simulink model "Pendule_TrueTime_SA"  (R2020a)
settings: Solver=ode45  StartTime=0.0  StopTime=30  RelTol=1e-3  EnableMultiTasking=on
libraries: truetime x3
settings Model: ExtModeAutoUpdateStatusClock=off  Creator=anton  LastModifiedBy=Pierre
settings DataIOCC: LimitDataPoints=on  SaveFormat=Array  SignalLoggingSaveFormat=ModelDataLogs  ReturnWorkspaceOutputs=off
settings OptimizationCC: BooleanDataType=off  LifeSpan=inf
settings DebuggingCC: SaveWithParameterizedLinksMsg=none  UnderspecifiedInitializationDetection=Classic  MergeDetectMultiDrivingBlocksExec=none  SignalResolutionControl=TryResolveAllWithWarning  MultiTaskDSMMsg=warning  MultiTaskCondExecSysMsg=none  FcnCallInpInsideContextMsg=warning  SFUnexpectedBacktrackingDiag=warning  SFNoUnconditionalDefaultTransitionDiag=warning  SFExecutionAtInitializationDiag=none  ArithmeticOperatorsInVariantConditions=warning
settings HardwareCC: ProdBitPerPointer=32  ProdBitPerSizeT=32  ProdBitPerPtrDiffT=32  ProdLargestAtomicFloat=None  ProdIntDivRoundTo=Undefined  ProdEndianess=Unspecified  ProdWordSize=32  ProdHWDeviceType=32-bit Generic  TargetUnknown=on
settings ModelReferenceCC: PropagateSignalLabelsOutOfModel=off
settings SFSimCC: SimUseLocalCustomCode=off  CustomCodeUndefinedFunction=UseInterfaceOnly
settings RTWCC: RTWUseLocalCustomCode=off
settings CodeAppCC: StateflowObjectComments=on
settings GRTTargetCC: TargetLangStandard=C89/C90 (ANSI)  CombineOutputUpdateFcns=off  GRTInterface=on
settings ConfigComp: CovMetricSettings=dw  CovHtmlReporting=on  CovSaveCumulativeToWorkspaceVar=on  CovSaveSingleToWorkspaceVar=on  CovExternalEMLEnable=off

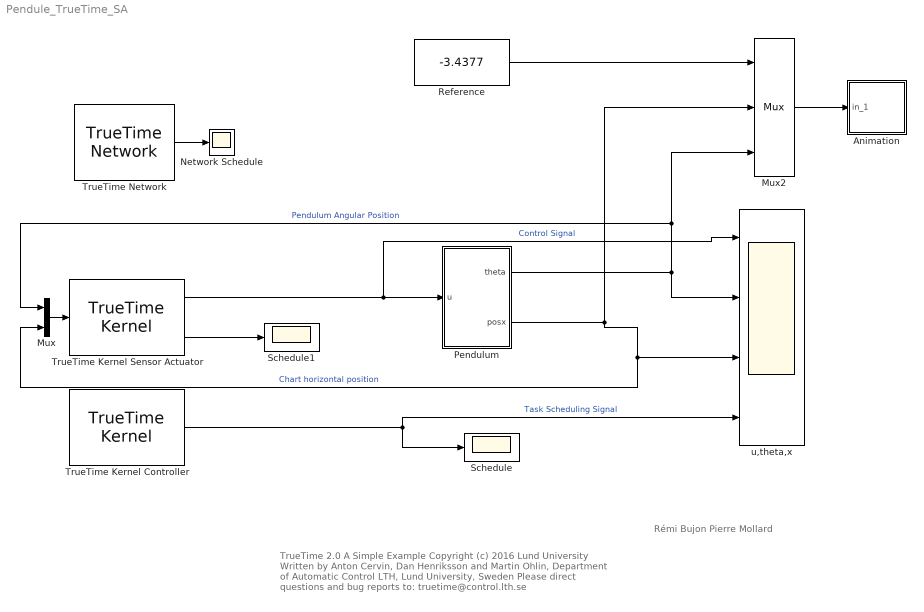
== system Pendule_TrueTime_SA ==
  note: TrueTime 2.0  A Simple Example
      | Copyright (c) 2016 Lund University
      | Written by Anton Cervin, Dan Henriksson and Martin Ohlin,
      | Department of Automatic Control LTH, Lund University, Sweden
      | Please direct questions and bug reports to: truetime@control.lth.se
  note: Rémi Bujon
      | Pierre Mollard
  Animation : Subsystem  mask(Pendulum plot){RefBlock=Reference}
      mask prompts: RefBlock "DC reference signal block name:"
      mask help: Pendulum plot
      mask Help: Pendulum animation function using Handle graphics.
      mask Display: plot([-10 10],[0 0],[-2 -2 2 2],[0 1 1 0],[0 3],[1 5])
  Mux : Mux  Inputs=2
  Mux2 : Mux  Inputs=3
  Network Schedule : Scope
  Pendulum : Subsystem
  Reference : Constant  Value=-3.4377
  Schedule : Scope
  Schedule1 : Scope
  TrueTime Kernel Controller : truetime/TrueTime Kernel  sfun=Controller_Init  args=0  ninputsoutputs=[0 0]  ntriggers=0  trigtype=falling  nwnodenbr=[2]  clockoffsetdrift=[0 0]  schedoutput=on  battery=off  poweroutput=off  label=1: 2
  TrueTime Kernel Sensor Actuator : truetime/TrueTime Kernel  sfun=Sensor_Actuator_Init  args=0  ninputsoutputs=[2 1]  ntriggers=0  trigtype=falling  nwnodenbr=[1]  clockoffsetdrift=[0 0]  schedoutput=on  battery=off  poweroutput=off  label=1: 1
  TrueTime Network : truetime/TrueTime Network  nwtype=CSMA/CD (Ethernet)  nwnbr=1  nnodes=2  rate=80000  minsize=80  lossprob=0  seed=0  bandwidths=[0.5 0.25 0.25]  slotsize=80  schedule=[1 2 1 3]  memsize=80000  buftype=Common buffer  overflow=Retransmit  dynSchedule=[]  miniSlotSize=40  NIT=0  QSortMode=FIFO  sync=0  irtSchedule=0  nrtLength=0  nodeGraph=0  scheduleoutput=on
  u,theta,x : Scope  NumInputPorts=4
  wires:
  TrueTime Kernel Controller/1 -> Schedule/1, u,theta,x/4  "Task Scheduling Signal"
  TrueTime Kernel Sensor Actuator/1 -> Pendulum/1(u), u,theta,x/1  "Control Signal"
  Pendulum/1(theta) -> Mux2/3, Mux/1, u,theta,x/2  "Pendulum Angular Position"
  Pendulum/2(posx) -> Mux/2, u,theta,x/3, Mux2/2  "Chart horizontal position"
  Reference/1 -> Mux2/1
  Mux2/1 -> Animation/1(in_1)
  Mux/1 -> TrueTime Kernel Sensor Actuator/1
  TrueTime Kernel Sensor Actuator/2 -> Schedule1/1
  TrueTime Network/1 -> Network Schedule/1

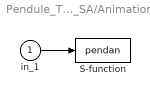
== system Pendule_TrueTime_SA/Animation ==
  in_1 : Inport
  S-function : S-Function  FunctionName=pendan  Parameters=RefBlock  SFunctionDeploymentMode=off  EnableBusSupport=off
      settings: DeleteFcn=pendan([],[],[],'DeleteBlock');
  wires:
  in_1/1 -> S-function/1

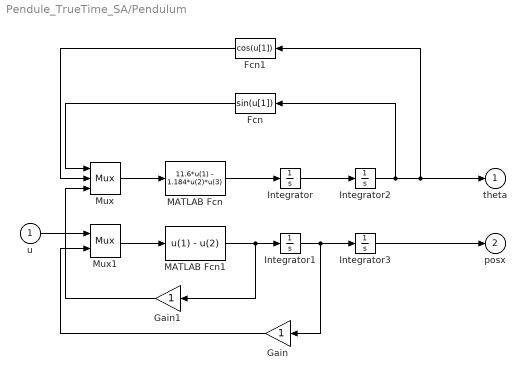
== system Pendule_TrueTime_SA/Pendulum ==
  u : Inport
  Fcn : Fcn
  Fcn1 : Fcn  Expr=cos(u[1])
  Gain : Gain  SaturateOnIntegerOverflow=on  OutDataTypeStr=Inherit: Same as input  ParamDataTypeStr=Inherit: Same as input
  Gain1 : Gain  SaturateOnIntegerOverflow=on  OutDataTypeStr=Inherit: Same as input  ParamDataTypeStr=Inherit: Same as input
  Integrator : Integrator
  Integrator1 : Integrator
  Integrator2 : Integrator  InitialCondition=0.1
  Integrator3 : Integrator
  MATLAB Fcn : MATLABFcn  MATLABFcn=11.6*u(1) - 1.184*u(2)*u(3)  OutputDimensions=1
  MATLAB Fcn1 : MATLABFcn  MATLABFcn=u(1) - u(2)  OutputDimensions=1
  Mux : Mux  Inputs=3
  Mux1 : Mux  Inputs=2
  theta : Outport  VectorParamsAs1DForOutWhenUnconnected=off
  posx : Outport  Port=2  VectorParamsAs1DForOutWhenUnconnected=off
  wires:
  Fcn1/1 -> Mux/2
  Integrator1/1 -> Gain/1, Integrator3/1
  Integrator3/1 -> posx/1
  Integrator/1 -> Integrator2/1
  Gain1/1 -> Mux/3
  Gain/1 -> Mux1/2
  MATLAB Fcn1/1 -> Gain1/1, Integrator1/1
  Integrator2/1 -> theta/1, Fcn1/1, Fcn/1
  MATLAB Fcn/1 -> Integrator/1
  Mux/1 -> MATLAB Fcn/1
  u/1 -> Mux1/1
  Mux1/1 -> MATLAB Fcn1/1
  Fcn/1 -> Mux/1
